simulink model "HopfOscillator_Simplelearning"  (R2019b)
settings: Solver=VariableStepAuto  StartTime=0.0  StopTime=3000  RelTol=1e-3
values from neighbouring files (symbols this model uses):
  i = zeros(1,3); i(1:N_osc) = 1    [PoolofAdaptiveOscillatorsThree.m]
  mu = 1    [SimplelearningExample.m]
settings Model: Creator=dell  LastModifiedBy=dell

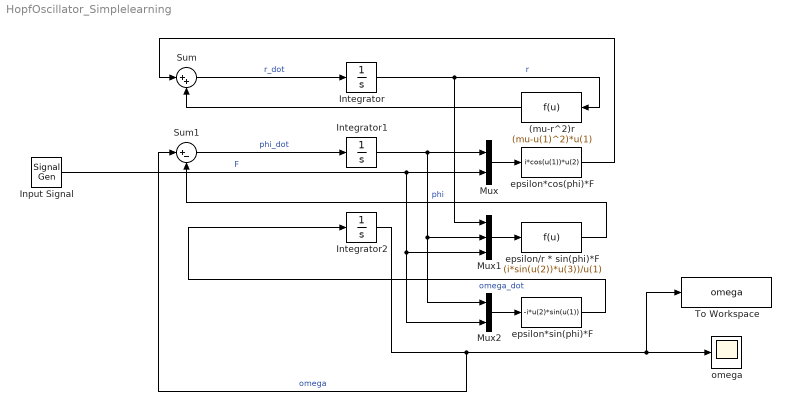
== system HopfOscillator_Simplelearning ==
  (mu-r^2)r : Fcn  Expr=(mu-u(1)^2)*u(1)
  Input Signal : SignalGenerator  Frequency=30  Units=rad/sec
  Integrator : Integrator  InitialCondition=1
  Integrator1 : Integrator
  Integrator2 : Integrator  InitialCondition=40
  Mux : Mux  Inputs=2
  Mux1 : Mux  Inputs=3
  Mux2 : Mux  Inputs=2
  Sum : Sum  Inputs=|++
  Sum1 : Sum  Inputs=|+-
  To Workspace : ToWorkspace  VariableName=omega  SaveFormat=Timeseries  SampleTime=-1
  epsilon*cos(phi)*F : Fcn  Expr=i*cos(u(1))*u(2)
  epsilon*sin(phi)*F : Fcn  Expr=-i*u(2)*sin(u(1))
  epsilon/r * sin(phi)*F : Fcn  Expr=(i*sin(u(2))*u(3))/u(1)
  "omega " : Scope
  wires:
  Integrator/1 -> (mu-r^2)r/1, Mux1/1  "r"
  Input Signal/1 -> Mux2/2, Mux1/3, Mux/2  "F"
  Integrator1/1 -> Mux1/2, Mux2/1, Mux/1  "phi"
  epsilon*sin(phi)*F/1 -> Integrator2/1  "omega_dot"
  Mux2/1 -> epsilon*sin(phi)*F/1
  Mux1/1 -> epsilon/r * sin(phi)*F/1
  epsilon*cos(phi)*F/1 -> Sum/1
  Integrator2/1 -> Sum1/1, To Workspace/1, "omega "/1  "omega"
  Sum1/1 -> Integrator1/1  "phi_dot"
  Sum/1 -> Integrator/1  "r_dot"
  epsilon/r * sin(phi)*F/1 -> Sum1/2
  (mu-r^2)r/1 -> Sum/2
  Mux/1 -> epsilon*cos(phi)*F/1
